simulink model "NPC_DC_5L_N2"  (R2017b)
settings: Solver=VariableStepAuto  StartTime=0.0  StopTime=30  MaxStep=1e-4  RelTol=1e-3
InitFcn:
  | mex DC_5L_MPC_RL_N2.c
libraries: powerlib x69
settings Model: Creator=alfonso  LastModifiedBy=alfonso

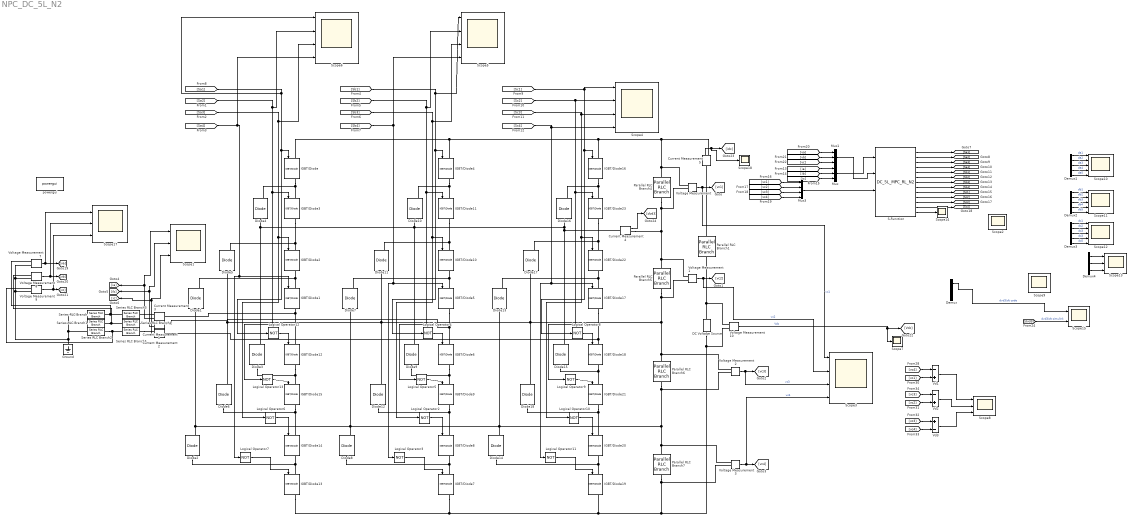
== system NPC_DC_5L_N2 ==
  Current Measurement{1..5} (5 alike) : powerlib/Measurements/Current Measurement  PhasorSimulation=off  OutputType=Complex  PSBequivalent=0
  DC Voltage Source : powerlib/Electrical Sources/DC Voltage Source  Amplitude=700  Measurements=None
  Demux : Demux  Outputs=3
  Demux1 : Demux  Outputs=5
  Demux2 : Demux  Outputs=5
  Demux3 : Demux  Outputs=5
  Demux4 : Demux  Outputs=3
  Diode{1..18} (18 alike) : powerlib/Power Electronics/Diode  Ron=0.001  Lon=0  Vf=0.8  IC=0  UseSnubber=0  Rs=500  Cs=250e-9  Measurements=on
  Ground : powerlib/Elements/Ground  LConnTagsString=a
  IGBT/Diode{,1..23} (24 alike) : powerlib/Power Electronics/IGBT//Diode  Ron=1e-3  Rs=1e5  Cs=inf  Measurements=on
  Logical Operator{2..13} (12 alike) : Logic  Operator=NOT  AllPortsSameDT=off  OutDataTypeStr=boolean
  Mux : Mux  Inputs=3
  Mux1 : Mux  Inputs=3
  Mux3 : Mux
  Parallel RLC Branch1 : powerlib/Elements/Parallel RLC Branch  LConnTagsString=a  RConnTagsString=__new0  BranchType=R  Resistance=1e-3  Inductance=0  SetiL0=off  InitialCurrent=0  Capacitance=3.3e-3  Setx0=off  InitialVoltage=0  Measurements=None
  Parallel RLC Branch{4..7} (4 alike) : powerlib/Elements/Parallel RLC Branch  LConnTagsString=a  RConnTagsString=__new0  BranchType=C  Resistance=0  Inductance=0  SetiL0=off  InitialCurrent=0  Capacitance=19.8e-3  Setx0=on  InitialVoltage=700/4  Measurements=None
  S-Function : S-Function  FunctionName=DC_5L_MPC_RL_N2  SFunctionDeploymentMode=off  EnableBusSupport=off
  Scope{1..2,8,13,17} (5 alike) : Scope  NumInputPorts=3
  Scope10 : Scope  NumInputPorts=5
  Scope11 : Scope  NumInputPorts=5
  Scope12 : Scope  NumInputPorts=5
  Scope14 : Scope
  Scope15 : Scope  NumInputPorts=2
  Scope18 : Scope
  Scope{3..6} (4 alike) : Scope  NumInputPorts=4
  Scope7 : Scope
  Scope9 : Scope  NumInputPorts=2
  Series RLC Branch : powerlib/Elements/Series RLC Branch  LConnTagsString=__new0  RConnTagsString=__new0  BranchType=R  Resistance=240  Inductance=2e-3  SetiL0=off  InitialCurrent=0  Capacitance=1e-6  Setx0=off  InitialVoltage=0  Measurements=None
  Series RLC Branch1 : powerlib/Elements/Series RLC Branch  LConnTagsString=__new0  RConnTagsString=__new0  BranchType=R  Resistance=240  Inductance=2e-3  SetiL0=off  InitialCurrent=0  Capacitance=1e-6  Setx0=off  InitialVoltage=0  Measurements=None
  Series RLC Branch2 : powerlib/Elements/Series RLC Branch  LConnTagsString=__new0  RConnTagsString=__new0  BranchType=R  Resistance=240  Inductance=2e-3  SetiL0=off  InitialCurrent=0  Capacitance=1e-6  Setx0=off  InitialVoltage=0  Measurements=None
  Series RLC Branch3 : powerlib/Elements/Series RLC Branch  LConnTagsString=__new0  RConnTagsString=__new0  BranchType=L  Resistance=240  Inductance=2e-3  SetiL0=off  InitialCurrent=0  Capacitance=1e-6  Setx0=off  InitialVoltage=0  Measurements=None
  Series RLC Branch4 : powerlib/Elements/Series RLC Branch  LConnTagsString=__new0  RConnTagsString=__new0  BranchType=L  Resistance=240  Inductance=2e-3  SetiL0=off  InitialCurrent=0  Capacitance=1e-6  Setx0=off  InitialVoltage=0  Measurements=None
  Series RLC Branch5 : powerlib/Elements/Series RLC Branch  LConnTagsString=__new0  RConnTagsString=__new0  BranchType=L  Resistance=240  Inductance=2e-3  SetiL0=off  InitialCurrent=0  Capacitance=1e-6  Setx0=off  InitialVoltage=0  Measurements=None
  Vd1 : Sum  Inputs=-+
  Vd2 : Sum  Inputs=-+
  Vd3 : Sum  Inputs=+-
  Voltage Measurement{,1..3,7..10} (8 alike) : powerlib/Measurements/Voltage Measurement  PhasorSimulation=off  OutputType=Complex  PSBequivalent=0
  powergui : powerlib/powergui  Priority=1  SimulationMode=Continuous  SampleTime=50e-6  frequency=60  Iterations=50  frequencyindice=0  Pbase=100e6  ErrMax=1e-4  UnitsV=kV  UnitsW=MW  buscounter=0  FunctionMessages=off  echomessages=off  EnableUseOfTLC=off  CurrentSourceSwitches=off  DisableSnubberDevices=off  DisableRonSwitches=off  DisableVfSwitches=off  DisplayEquations=off  SolverType=Tustin/Backward Euler (TBE)  Interpol=off  ExternalGateDelay=off  methode=off  Ts=100  x0status=blocks  SPID=on  SwTol=0  HookPort=off  RestoreLinks=warning  ResistiveCurrentMeasurement=off  Frange=[0:2:500]  Ylog=off  Xlog=on  ShowGrid=off  save=off  variable=ZData  structure=0  ZoomFFT=off  StartTime=0.0  cycles=1  DisplayStyle=1  fundamental=60  FreqAxis=off  MaxFrequency=1000  frequencyindicesteady=1  RmsSteady=1  display=off
  wires:
  [Sc2] -> Scope4/2, IGBT/Diode23/1, Logical Operator9/1
  [Sc3] -> Scope4/3, Logical Operator10/1, IGBT/Diode22/1
  [Sc4] -> Scope4/4, IGBT/Diode17/1, Logical Operator11/1
  Logical Operator11/1 -> IGBT/Diode19/1
  Logical Operator10/1 -> IGBT/Diode20/1
  Logical Operator9/1 -> IGBT/Diode21/1
  Logical Operator8/1 -> IGBT/Diode18/1
  Logical Operator3/1 -> IGBT/Diode7/1
  Logical Operator4/1 -> IGBT/Diode6/1
  Logical Operator5/1 -> IGBT/Diode9/1
  Logical Operator2/1 -> IGBT/Diode8/1
  Logical Operator6/1 -> IGBT/Diode14/1
  Logical Operator7/1 -> IGBT/Diode13/1
  Logical Operator13/1 -> IGBT/Diode15/1
  Logical Operator12/1 -> IGBT/Diode12/1
  Voltage Measurement/1 -> Scope3/1, [vc1]  "vc1"
  Voltage Measurement1/1 -> Scope3/2, [vc2]  "vc2"
  Voltage Measurement2/1 -> Scope3/3, [vc3]  "vc3"
  Voltage Measurement3/1 -> Scope3/4, [vc4]  "vc4"
  [ia] -> Mux/1
  [ib] -> Mux/2
  [ic] -> Mux/3
  S-Function/12 -> [Sc4]
  S-Function/11 -> [Sc3]
  S-Function/10 -> [Sc2]
  S-Function/9 -> [Sc1]
  S-Function/8 -> [Sb4]
  S-Function/7 -> [Sb3]
  S-Function/6 -> [Sb2]
  S-Function/5 -> [Sb1]
  S-Function/4 -> [Sa4]
  S-Function/1 -> [Sa1]
  S-Function/2 -> [Sa2]
  S-Function/3 -> [Sa3]
  [Sc1] -> Scope4/1, IGBT/Diode16/1, Logical Operator8/1
  [vc] -> Mux1/3
  [vb] -> Mux1/2
  [va] -> Mux1/1
  [Sb2] -> Scope5/2, IGBT/Diode11/1, Logical Operator5/1
  [Sb3] -> Scope5/3, IGBT/Diode10/1, Logical Operator2/1
  [Sb1] -> Scope5/1, IGBT/Diode4/1, Logical Operator4/1
  [Sb4] -> Logical Operator3/1, IGBT/Diode5/1, Scope5/4
  [Sa3] -> Scope6/3, IGBT/Diode2/1, Logical Operator6/1
  [Sa2] -> Scope6/2, IGBT/Diode3/1, Logical Operator13/1
  [Sa4] -> Scope6/4, Logical Operator7/1, IGBT/Diode1/1
  [Sa1] -> Scope6/1, IGBT/Diode/1, Logical Operator12/1
  Voltage Measurement10/1 -> Scope7/1, [Vdc]  "Vdc"
  Current Measurement3/1 -> [ia], Scope1/1
  Current Measurement2/1 -> [ic], Scope1/3
  Mux1/1 -> S-Function/2
  Demux/1 -> Scope15/1  "dvd3/dt code"
  Demux1/1 -> Scope10/1  "da1"
  Demux1/2 -> Scope10/2  "da2"
  Demux1/3 -> Scope10/3  "da3"
  Demux1/4 -> Scope10/4  "da4"
  Demux2/4 -> Scope11/4  "db4"
  Demux2/2 -> Scope11/2  "db2"
  Demux2/3 -> Scope11/3  "db3"
  Demux2/1 -> Scope11/1  "db1"
  Demux3/4 -> Scope12/4  "dc3"
  Demux3/2 -> Scope12/2  "dc2"
  Demux3/3 -> Scope12/3  "dc3"
  Demux3/1 -> Scope12/1  "dc1"
  Demux4/1 -> Scope13/1
  Demux4/2 -> Scope13/2
  Demux4/3 -> Scope13/3
  Demux3/5 -> Scope12/5  "dc5"
  Demux2/5 -> Scope11/5  "db5"
  Demux1/5 -> Scope10/5  "da5"
  Current Measurement1/1 -> [ib], Scope1/2
  Voltage Measurement7/1 -> Scope17/1, [va]
  Voltage Measurement9/1 -> Scope17/3, [vc]
  Voltage Measurement8/1 -> Scope17/2, [vb]
  Mux/1 -> S-Function/1
  Vd2/1 -> Scope8/2
  [vc1] -> Vd1/2
  Vd1/1 -> Scope8/1
  [vc2] -> Vd2/2
  [vc3] -> Vd3/1
  Vd3/1 -> Scope8/3
  [vc4] -> Vd1/1
  [vc3] -> Vd2/1
  [vc4] -> Vd3/2
  Current Measurement4/1 -> [dvd3]
  [dvd3] -> Scope15/2  "dvd3/dt simulink"
  [vc2] -> Mux3/2
  [vc3] -> Mux3/3
  [vc1] -> Mux3/1
  Mux3/1 -> S-Function/3
  [vc4] -> Mux3/4
  Current Measurement5/1 -> Scope18/1, [idc]
  S-Function/13 -> Scope14/1
  connections:
  IGBT/Diode/RConn1 -- Diode4/RConn1 -- IGBT/Diode3/LConn1
  IGBT/Diode1/LConn1 -- Diode1/RConn1 -- IGBT/Diode2/RConn1
  IGBT/Diode3/RConn1 -- Diode5/RConn1 -- IGBT/Diode2/LConn1
  IGBT/Diode15/RConn1 -- IGBT/Diode14/LConn1 -- Diode6/LConn1
  IGBT/Diode13/LConn1 -- Diode2/LConn1 -- IGBT/Diode14/RConn1
  IGBT/Diode12/RConn1 -- Diode3/LConn1 -- IGBT/Diode15/LConn1
  IGBT/Diode1/RConn1 -- Current Measurement3/LConn1 -- IGBT/Diode12/LConn1
  Diode15/RConn1 -- Diode16/LConn1 -- Diode4/LConn1 -- Diode3/RConn1 -- Diode10/LConn1 -- Diode9/RConn1 -- Current Measurement4/LConn1
  Diode6/RConn1 -- Voltage Measurement2/LConn1 -- Parallel RLC Branch6/LConn1 -- Parallel RLC Branch5/RConn1 -- Voltage Measurement1/LConn2 -- Diode18/RConn1 -- Diode17/LConn1 -- Diode11/LConn1 -- Diode12/RConn1 -- Diode5/LConn1
  IGBT/Diode11/RConn1 -- Diode11/RConn1 -- IGBT/Diode10/LConn1
  IGBT/Diode5/LConn1 -- Diode7/RConn1 -- IGBT/Diode10/RConn1
  IGBT/Diode9/RConn1 -- IGBT/Diode8/LConn1 -- Diode12/LConn1
  IGBT/Diode7/LConn1 -- Diode8/LConn1 -- IGBT/Diode8/RConn1
  IGBT/Diode4/RConn1 -- Diode10/RConn1 -- IGBT/Diode11/LConn1
  IGBT/Diode6/RConn1 -- Diode9/LConn1 -- IGBT/Diode9/LConn1
  IGBT/Diode5/RConn1 -- Current Measurement1/LConn1 -- IGBT/Diode6/LConn1
  IGBT/Diode23/RConn1 -- Diode17/RConn1 -- IGBT/Diode22/LConn1
  IGBT/Diode17/LConn1 -- Diode13/RConn1 -- IGBT/Diode22/RConn1
  IGBT/Diode21/RConn1 -- IGBT/Diode20/LConn1 -- Diode18/LConn1
  IGBT/Diode19/LConn1 -- Diode14/LConn1 -- IGBT/Diode20/RConn1
  IGBT/Diode16/RConn1 -- Diode16/RConn1 -- IGBT/Diode23/LConn1
  IGBT/Diode18/RConn1 -- Diode15/LConn1 -- IGBT/Diode21/LConn1
  IGBT/Diode17/RConn1 -- Current Measurement2/LConn1 -- IGBT/Diode18/LConn1
  Parallel RLC Branch7/RConn1 -- Voltage Measurement3/LConn2 -- DC Voltage Source/LConn1 -- Voltage Measurement10/LConn2 -- IGBT/Diode13/RConn1 -- IGBT/Diode7/RConn1 -- IGBT/Diode19/RConn1
  Series RLC Branch2/LConn1 -- Voltage Measurement9/LConn1 -- Series RLC Branch5/RConn1
  Series RLC Branch1/LConn1 -- Voltage Measurement8/LConn1 -- Series RLC Branch4/RConn1
  Voltage Measurement7/LConn1 -- Series RLC Branch3/RConn1 -- Series RLC Branch/LConn1
  Series RLC Branch2/RConn1 -- Series RLC Branch/RConn1 -- Series RLC Branch1/RConn1 -- Voltage Measurement7/LConn2 -- Voltage Measurement8/LConn2 -- Voltage Measurement9/LConn2 -- Ground/LConn1
  Voltage Measurement10/LConn1 -- Parallel RLC Branch1/RConn1 -- DC Voltage Source/RConn1
  IGBT/Diode/LConn1 -- Current Measurement5/RConn1 -- Voltage Measurement/LConn1 -- Parallel RLC Branch4/LConn1 -- IGBT/Diode16/LConn1 -- IGBT/Diode4/LConn1
  Parallel RLC Branch1/LConn1 -- Current Measurement5/LConn1
  Parallel RLC Branch4/RConn1 -- Voltage Measurement1/LConn1 -- Parallel RLC Branch5/LConn1 -- Current Measurement4/RConn1 -- Voltage Measurement/LConn2
  Diode2/RConn1 -- Parallel RLC Branch7/LConn1 -- Voltage Measurement3/LConn1 -- Voltage Measurement2/LConn2 -- Parallel RLC Branch6/RConn1 -- Diode14/RConn1 -- Diode13/LConn1 -- Diode7/LConn1 -- Diode8/RConn1 -- Diode1/LConn1
  Series RLC Branch5/LConn1 -- Current Measurement2/RConn1
  Series RLC Branch4/LConn1 -- Current Measurement1/RConn1
  Current Measurement3/RConn1 -- Series RLC Branch3/LConn1
